simulink model "scon_L8_1ponto5_simulink"  (R2024a)
settings: Solver=VariableStepAuto  StartTime=0.0  StopTime=10.0  RelTol=1e-3
values from neighbouring files (symbols this model uses):
  A = [0, 1, 0; 0, 0, 1; 0, -16, -10]    [scon2_L8_1ponto5.m]
  B = [0; 0; 120]    [scon2_L8_1ponto5.m]
  K = acker(A, B, J)    [scon2_L8_1ponto5.m]
settings Model: Creator=Carlos Augusto  LastModifiedBy=Carlos Augusto

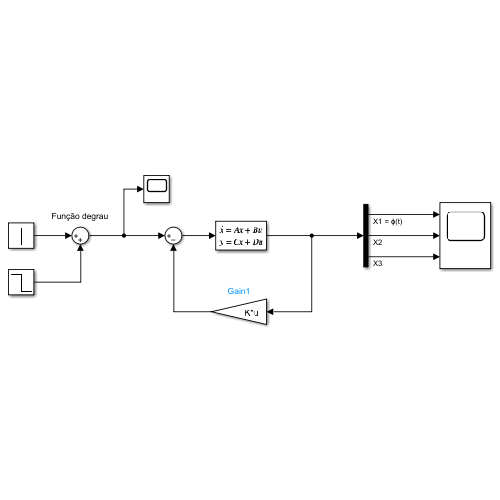
[thumbnail: Simulink's stored preview of the top-level diagram]
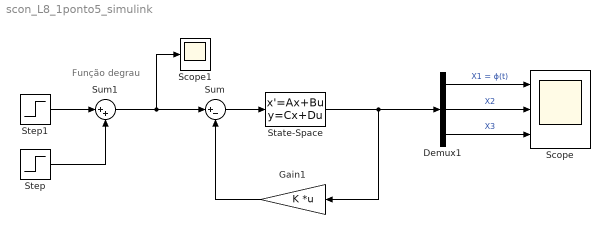
== system scon_L8_1ponto5_simulink ==
  note: Função degrau
  Demux1 : Demux  Outputs=3
  Gain1 : Gain  Gain=K  Multiplication=Matrix(K*u)
  Scope : Scope  NumInputPorts=3
  Scope1 : Scope
  State-Space : StateSpace  A=A  B=B  C=eye(3)  D=zeros(3,1)  InitialCondition=0
  Step : Step  Time=1.1  After=-10  SampleTime=0
  Step1 : Step  After=10  SampleTime=0
  Sum : Sum  Inputs=|+-
  Sum1 : Sum  Inputs=|++
  wires:
  State-Space/1 -> Demux1/1, Gain1/1
  Demux1/1 -> Scope/1  "X1 = ϕ(t)"
  Demux1/3 -> Scope/3  "X3"
  Demux1/2 -> Scope/2  "X2"
  Sum/1 -> State-Space/1
  Gain1/1 -> Sum/2
  Step1/1 -> Sum1/1
  Step/1 -> Sum1/2
  Sum1/1 -> Sum/1, Scope1/1
